simulink model "q3_continuos_non_adaptive_controller"  (R2019a)
settings: Solver=VariableStepAuto  StartTime=0.0  StopTime=20  RelTol=1e-3
values from neighbouring files (symbols this model uses):
  gama = 15    [adaptive_control_workspace.m]
  K = 10    [adaptive_control_workspace.m]
  k1 = 10    [adaptive_control_workspace.m]
  k2 = 10    [adaptive_control_workspace.m]
  lamda_0 = 7    [adaptive_control_workspace.m]
  lamda_1 = 4    [adaptive_control_workspace.m]
  lamda_2 = 8.4    [adaptive_control_workspace.m]
  m = 10    [adaptive_control_workspace.m]
settings Model: Creator=ronil  LastModifiedBy=ronil

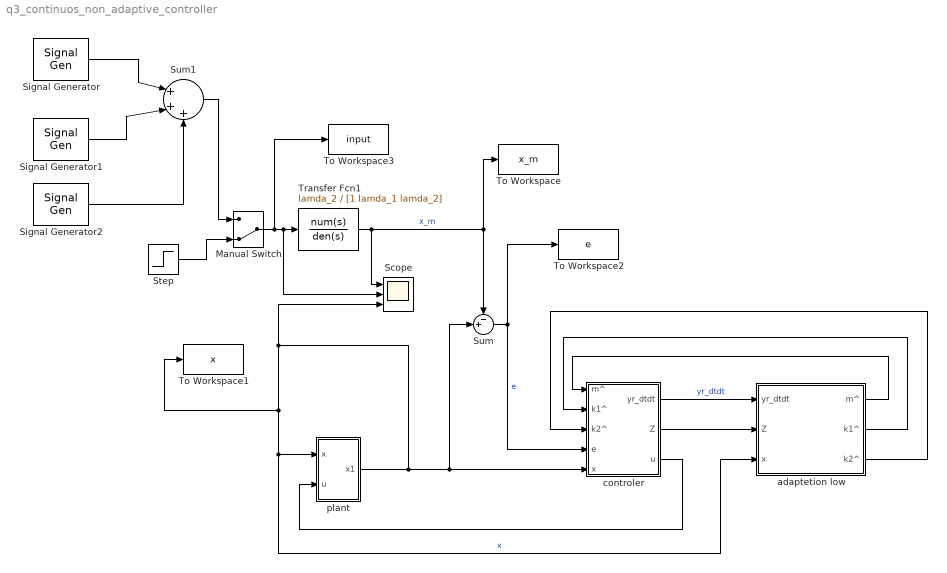
== system q3_continuos_non_adaptive_controller ==
  Manual Switch : ManualSwitch  CurrentSetting=0
  Scope : Scope  NumInputPorts=3
  Signal Generator : SignalGenerator  Amplitude=2  Frequency=0.4  Units=rad/sec
  Signal Generator1 : SignalGenerator  WaveForm=square  Amplitude=2  Frequency=0.5  Units=rad/sec
  Signal Generator2 : SignalGenerator  WaveForm=sawtooth  Frequency=0.3  Units=rad/sec
  Step : Step  SampleTime=0
  Sum : Sum  Inputs=-+|
  Sum1 : Sum  Inputs=|+++
  To Workspace : ToWorkspace  VariableName=x_m  SaveFormat=Timeseries  SampleTime=-1
  To Workspace1 : ToWorkspace  VariableName=x  SaveFormat=Timeseries  SampleTime=-1
  To Workspace2 : ToWorkspace  VariableName=e  SaveFormat=Timeseries  SampleTime=-1
  To Workspace3 : ToWorkspace  VariableName=input  SaveFormat=Timeseries  SampleTime=-1
  Transfer Fcn1 : TransferFcn  Numerator=lamda_2  Denominator=[1 lamda_1 lamda_2]
  adaptetion low : Subsystem
  controler : Subsystem
  plant : Subsystem
  wires:
  Transfer Fcn1/1 -> To Workspace/1, Sum/1, Scope/1  "x_m"
  plant/1(x1) -> Scope/3, plant/1(x), adaptetion low/3(x), To Workspace1/1, controler/5(x), Sum/2  "x"
  Signal Generator/1 -> Sum1/1
  controler/3(u) -> plant/2(u)
  Sum/1 -> To Workspace2/1, controler/4(e)  "e"
  controler/1(yr_dtdt) -> adaptetion low/1(yr_dtdt)  "yr_dtdt"
  controler/2(Z) -> adaptetion low/2(Z)
  adaptetion low/1(m^) -> controler/1(m^)
  adaptetion low/2(k1^) -> controler/2(k1^)
  Step/1 -> Manual Switch/2
  Signal Generator1/1 -> Sum1/2
  Signal Generator2/1 -> Sum1/3
  Sum1/1 -> Manual Switch/1
  Manual Switch/1 -> To Workspace3/1, Transfer Fcn1/1, Scope/2
  adaptetion low/3(k2^) -> controler/3(k2^)

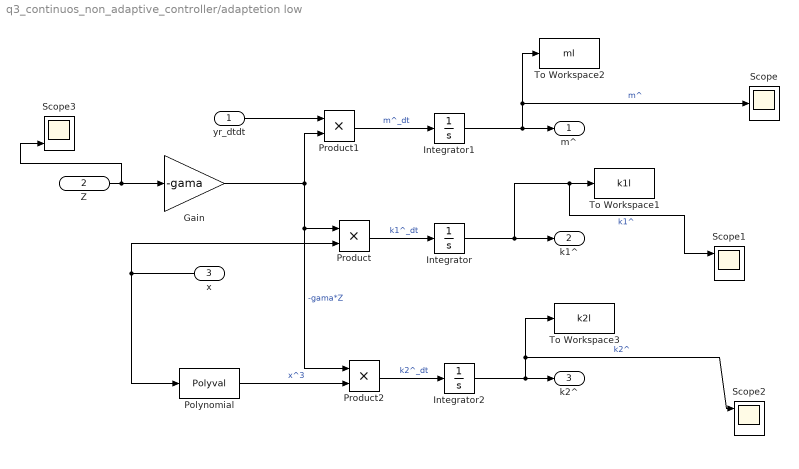
== system q3_continuos_non_adaptive_controller/adaptetion low ==
  yr_dtdt : Inport
  Z : Inport  Port=2
  x : Inport  Port=3
  Gain : Gain  Gain=-gama
  Integrator : Integrator
  Integrator1 : Integrator
  Integrator2 : Integrator
  Polynomial : Polyval  Coefs=[1 0 0 0]
  Product : Product
  Product1 : Product
  Product2 : Product
  Scope{,1..3} (4 alike) : Scope  NumInputPorts=3
  To Workspace1 : ToWorkspace  VariableName=k1l  SaveFormat=Timeseries  SampleTime=-1
  To Workspace2 : ToWorkspace  VariableName=ml  SaveFormat=Timeseries  SampleTime=-1
  To Workspace3 : ToWorkspace  VariableName=k2l  SaveFormat=Timeseries  SampleTime=-1
  m^ : Outport
  k1^ : Outport  Port=2
  k2^ : Outport  Port=3
  wires:
  Polynomial/1 -> Product2/2  "x^3"
  Gain/1 -> Product1/2, Product2/1, Product/1  "-gama*Z"
  Integrator/1 -> Scope1/1, To Workspace1/1, k1^/1  "k1^"
  Product/1 -> Integrator/1  "k1^_dt"
  Product2/1 -> Integrator2/1  "k2^_dt"
  Product1/1 -> Integrator1/1  "m^_dt"
  Integrator1/1 -> Scope/2, To Workspace2/1, m^/1  "m^"
  Z/1 -> Scope3/3, Gain/1
  x/1 -> Polynomial/1, Product/2
  yr_dtdt/1 -> Product1/1
  Integrator2/1 -> To Workspace3/1, Scope2/1, k2^/1  "k2^"

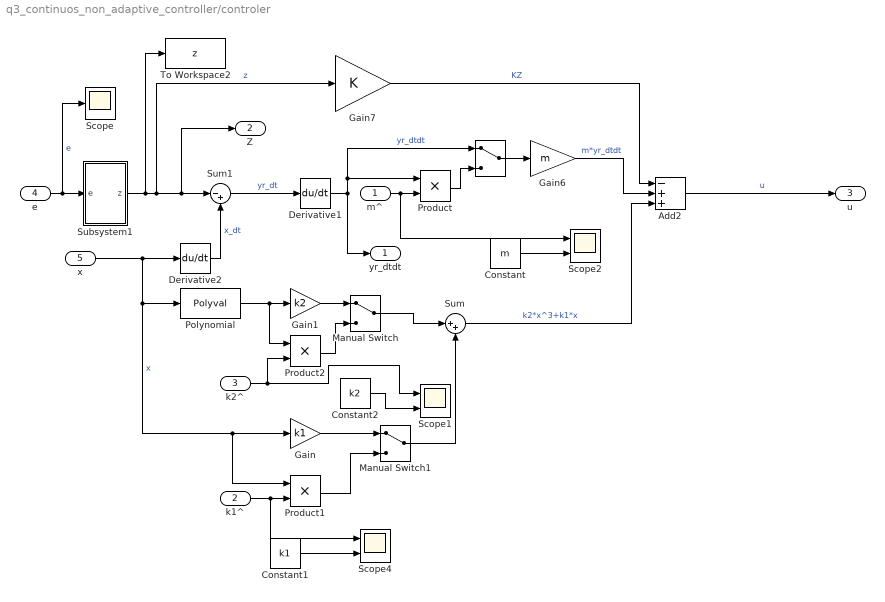
== system q3_continuos_non_adaptive_controller/controler ==
  m^ : Inport
  k1^ : Inport  Port=2
  k2^ : Inport  Port=3
  e : Inport  Port=4
  x : Inport  Port=5
  " " : ManualSwitch
  Add2 : Sum  Inputs=-++
  Constant : Constant  Value=m
  Constant1 : Constant  Value=k1
  Constant2 : Constant  Value=k2
  Derivative1 : Derivative
  Derivative2 : Derivative
  Gain : Gain  Gain=k1
  Gain1 : Gain  Gain=k2
  Gain6 : Gain  Gain=m
  Gain7 : Gain  Gain=K
  Manual Switch : ManualSwitch
  Manual Switch1 : ManualSwitch
  Polynomial : Polyval  Coefs=[1 0 0 0]
  Product : Product
  Product1 : Product
  Product2 : Product
  Scope : Scope
  Scope1 : Scope  NumInputPorts=2
  Scope2 : Scope  NumInputPorts=2
  Scope4 : Scope  NumInputPorts=2
  Subsystem1 : Subsystem
  Sum : Sum  Inputs=|++
  Sum1 : Sum  Inputs=|-+
  To Workspace2 : ToWorkspace  VariableName=z  SaveFormat=Timeseries  SampleTime=-1
  yr_dtdt : Outport
  Z : Outport  Port=2
  u : Outport  Port=3
  wires:
  Gain6/1 -> Add2/2  "m*yr_dtdt"
  Sum1/1 -> Derivative1/1  "yr_dt"
  Subsystem1/1(z) -> To Workspace2/1, Gain7/1, Z/1, Sum1/1  "z"
  Derivative1/1 -> " "/1, Product/1, yr_dtdt/1  "yr_dtdt"
  Gain7/1 -> Add2/1  "KZ"
  Sum/1 -> Add2/3  "k2*x^3+k1*x"
  Add2/1 -> u/1  "u"
  e/1 -> Scope/1, Subsystem1/1(e)  "e"
  x/1 -> Product1/1, Gain/1, Polynomial/1, Derivative2/1  "x"
  Derivative2/1 -> Sum1/2  "x_dt"
  Polynomial/1 -> Product2/1, Gain1/1
  Gain1/1 -> Manual Switch/1
  Gain/1 -> Manual Switch1/1
  Manual Switch/1 -> Sum/1
  k2^/1 -> Scope1/1, Product2/2
  Product2/1 -> Manual Switch/2
  k1^/1 -> Scope4/1, Product1/2
  Product1/1 -> Manual Switch1/2
  Manual Switch1/1 -> Sum/2
  m^/1 -> Scope2/1, Product/2
  " "/1 -> Gain6/1
  Product/1 -> " "/2
  Constant/1 -> Scope2/2
  Constant1/1 -> Scope4/2
  Constant2/1 -> Scope1/2

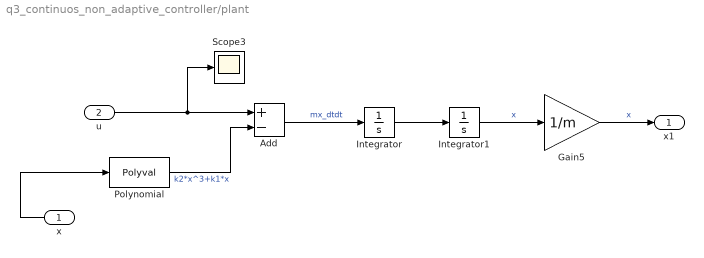
== system q3_continuos_non_adaptive_controller/plant ==
  x : Inport
  u : Inport  Port=2
  Add : Sum  Inputs=+-
  Gain5 : Gain  Gain=1/m
  Integrator : Integrator
  Integrator1 : Integrator
  Polynomial : Polyval  Coefs=[k2 0 k1 0]
  Scope3 : Scope
  x1 : Outport
  wires:
  Integrator/1 -> Integrator1/1
  Integrator1/1 -> Gain5/1  "x"
  Polynomial/1 -> Add/2  "k2*x^3+k1*x"
  x/1 -> Polynomial/1
  u/1 -> Add/1, Scope3/1
  Add/1 -> Integrator/1  "mx_dtdt"
  Gain5/1 -> x1/1  "x"

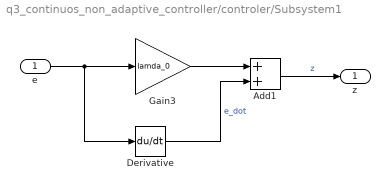
== system q3_continuos_non_adaptive_controller/controler/Subsystem1 ==
  e : Inport
  Add1 : Sum
  Derivative : Derivative
  Gain3 : Gain  Gain=lamda_0
  z : Outport
  wires:
  e/1 -> Derivative/1, Gain3/1
  Gain3/1 -> Add1/1
  Derivative/1 -> Add1/2  "e_dot"
  Add1/1 -> z/1  "z"
